simulink model "FIR_direct_ref_model"  (R2020a)
settings: Solver=VariableStepAuto  StartTime=0.0  StopTime=10.0  RelTol=1e-3
settings Model: Creator=Prateek  LastModifiedBy=Prateek
settings DataIOCC: SaveOutput=off  SaveTime=off

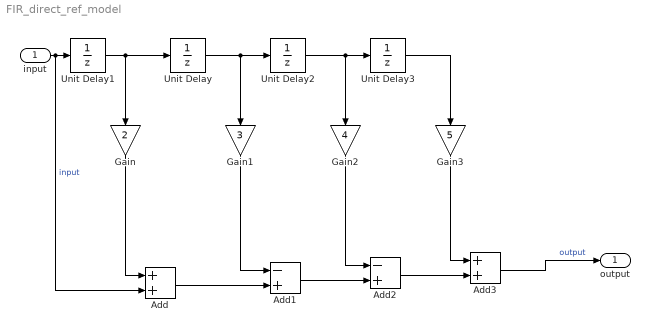
== system FIR_direct_ref_model ==
  input : Inport  OutDataTypeStr=double  PortDimensions=1  SampleTime=[0,1]
  Add : Sum
  Add1 : Sum  Inputs=-+
  Add2 : Sum  Inputs=-+
  Add3 : Sum
  Gain : Gain  Gain=2
  Gain1 : Gain  Gain=3
  Gain2 : Gain  Gain=4
  Gain3 : Gain  Gain=5
  Unit Delay{,1..3} (4 alike) : UnitDelay  SampleTime=-1  HasFrameUpgradeWarning=on
  output : Outport  OutDataTypeStr=double  PortDimensions=1  SampleTime=[0,1]
  wires:
  Add1/1 -> Add2/2
  Gain/1 -> Add/1
  Unit Delay1/1 -> Gain/1, Unit Delay/1
  Add/1 -> Add1/2
  Unit Delay/1 -> Unit Delay2/1, Gain1/1
  Add2/1 -> Add3/2
  Unit Delay2/1 -> Unit Delay3/1, Gain2/1
  Gain1/1 -> Add1/1
  Unit Delay3/1 -> Gain3/1
  Gain3/1 -> Add3/1
  Gain2/1 -> Add2/1
  input/1 -> Unit Delay1/1, Add/2  "input"
  Add3/1 -> output/1  "output"
